simulink model "tp4_2"  (R2024b)
settings: Solver=FixedStepAuto  StartTime=0.0  StopTime=500  FixedStep=0.1  RelTol=1e-3
values from neighbouring files (symbols this model uses):
  F_in = 0.0035    [codigo_profe.m]    (also in directo.m; directo2.m; discretization.m; efecto_integral.m)
  F_out_sin_k = a*sqrt(2*g)    [tp4_inicio.m]
  h_list = [0.2, 0.4, 0.6, 0.8]    [tp4_inicio.m]
  k_list = [0.05, 0.15, 0.30, 0.50, 0.90]    [directo.m]    (also in directo2.m; discretization.m; efecto_integral.m; indirecto.m)
  r_0 = 0.05    [codigo_profe.m]    (also in directo.m; directo2.m; discretization.m; efecto_integral.m)
  theta = 60    [codigo_profe.m]    (also in directo.m; directo2.m; discretization.m; efecto_integral.m)
undefined symbols (not defined in the file or in its folder): A, B, C, D
libraries: ctrlSharedLib x1, simulink x1
settings Model: Creator=trulscarlson  LastModifiedBy=trulscarlson
settings DebuggingCC: UnconnectedInputMsg=warning  UnconnectedOutputMsg=warning  UnconnectedLineMsg=warning
settings ModelReferenceCC: EnableRefExpFcnMdlSchedulingChecks=on
settings RTWCC: GPUComputeCapability=3.5  DLArmComputeVersion=19.05

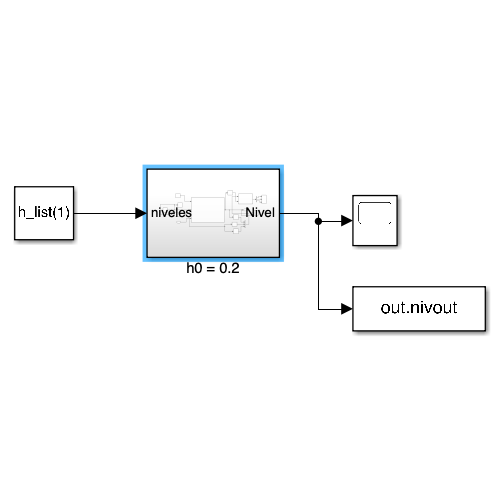
[thumbnail: Simulink's stored preview of the top-level diagram]
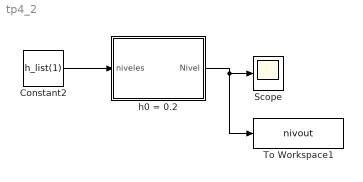
== system tp4_2 ==
  Constant2 : Constant  Value=h_list(1)
  Scope : Scope
  To Workspace1 : ToWorkspace  VariableName=nivout  SaveFormat=Timeseries  SampleTime=-1
  h0 = 0.2 : Subsystem
  wires:
  Constant2/1 -> h0 = 0.2/1(niveles)
  h0 = 0.2/1(Nivel) -> To Workspace1/1, Scope/1

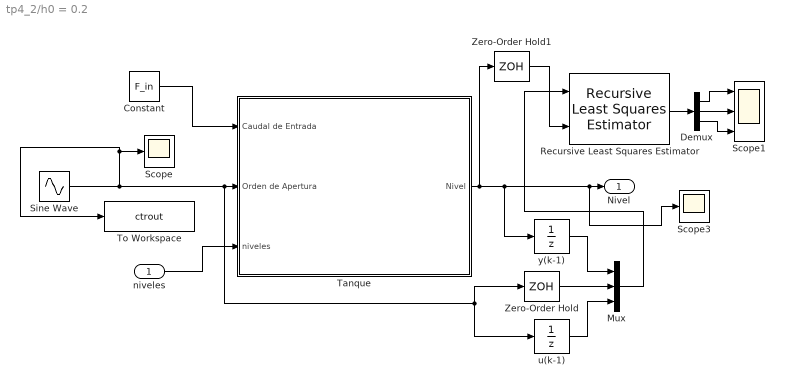
== system tp4_2/h0 = 0.2 ==
  niveles : Inport
  Constant : Constant  Value=F_in
  Demux : Demux  Outputs=3
  Mux : Mux  Inputs=3
  Recursive Least Squares Estimator : ctrlSharedLib/Recursive Least Squares Estimator  InitialEstimateSource=Internal  InitialParameterData=[0 0 0]  P0=1e5  InitialRegressors=0  InitialOutputs=0  History=Infinite  WindowLength=200  EstimationMethod=Forgetting Factor  AdaptationParameter=0.99  HasTimeVaryingAdaptationParameter=off  NormalizationBias=eps  OutputError=off  OutputP=off  AddEnablePort=off  InputProcessing=Sample-based  Ts=-1
      settings: LibrarySourceBlock=slident/Estimators/Recursive Least Squares Estimator
  Scope : Scope
  Scope1 : Scope  NumInputPorts=3
  Scope3 : Scope
  Sine Wave : Sin  Amplitude=0.2  Bias=k_list(1)  SampleTime=0
  Tanque : Subsystem
  To Workspace : ToWorkspace  VariableName=ctrout  SaveFormat=Timeseries  SampleTime=-1
  Zero-Order Hold : ZeroOrderHold  SampleTime=-1
  Zero-Order Hold1 : ZeroOrderHold  SampleTime=-1
  u(k-1) : UnitDelay  InitialCondition=k_list(1)  SampleTime=-1  HasFrameUpgradeWarning=on
  y(k-1) : UnitDelay  InitialCondition=h_list(1)  SampleTime=-1  HasFrameUpgradeWarning=on
  Nivel : Outport
  wires:
  niveles/1 -> Tanque/3(niveles)
  Constant/1 -> Tanque/1(Caudal de Entrada)
  Tanque/1(Nivel) -> Zero-Order Hold1/1, Scope3/1, Nivel/1, y(k-1)/1
  Sine Wave/1 -> Scope/1, To Workspace/1, u(k-1)/1, Zero-Order Hold/1, Tanque/2(Orden de Apertura)
  y(k-1)/1 -> Mux/1
  u(k-1)/1 -> Mux/3
  Mux/1 -> Recursive Least Squares Estimator/1
  Zero-Order Hold/1 -> Mux/2
  Zero-Order Hold1/1 -> Recursive Least Squares Estimator/2
  Recursive Least Squares Estimator/1 -> Demux/1
  Demux/1 -> Scope1/1
  Demux/2 -> Scope1/2
  Demux/3 -> Scope1/3

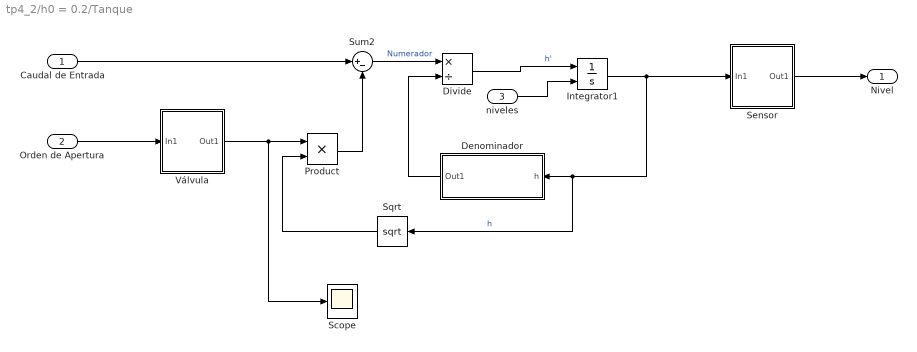
== system tp4_2/h0 = 0.2/Tanque ==
  Caudal de Entrada : Inport
  Orden de Apertura : Inport  Port=2
  niveles : Inport  Port=3
  Denominador : Subsystem
  Divide : Product  Inputs=*/
  Integrator1 : Integrator  InitialConditionSource=external  InitialCondition=h_list(5)
  Product : Product
  Scope : Scope
  Sensor : Subsystem
  Sqrt : Sqrt
  Sum2 : Sum  Inputs=|+-
  Válvula : Subsystem
  Nivel : Outport
  wires:
  Product/1 -> Sum2/2
  Divide/1 -> Integrator1/1  "h'"
  Denominador/1(Out1) -> Divide/2
  Integrator1/1 -> Sensor/1(In1), Sqrt/1, Denominador/1(h)  "h"
  Sum2/1 -> Divide/1  "Numerador"
  Sqrt/1 -> Product/2
  Caudal de Entrada/1 -> Sum2/1
  Orden de Apertura/1 -> Válvula/1(In1)
  Válvula/1(Out1) -> Product/1, Scope/1
  niveles/1 -> Integrator1/2
  Sensor/1(Out1) -> Nivel/1

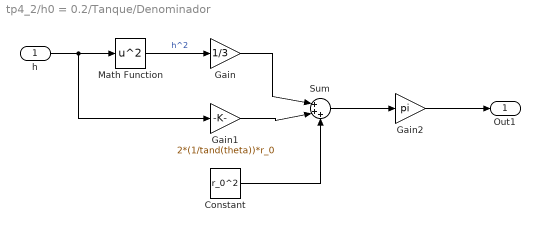
== system tp4_2/h0 = 0.2/Tanque/Denominador ==
  h : Inport
  Constant : Constant  Value=r_0^2
  Gain : Gain  Gain=1/3
  Gain1 : Gain  Gain=2*(1/tand(theta))*r_0
  Gain2 : Gain  Gain=pi
  Math Function : Math  Operator=square
  Sum : Sum  Inputs=|+++
  Out1 : Outport
  wires:
  h/1 -> Gain1/1, Math Function/1
  Math Function/1 -> Gain/1  "h^2"
  Gain/1 -> Sum/1
  Gain1/1 -> Sum/2
  Constant/1 -> Sum/3
  Sum/1 -> Gain2/1
  Gain2/1 -> Out1/1

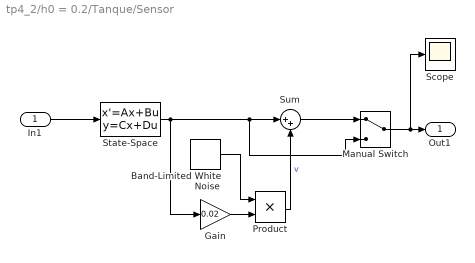
== system tp4_2/h0 = 0.2/Tanque/Sensor ==
  In1 : Inport
  Band-Limited White Noise : simulink/Sources/Band-Limited White Noise  Cov=[0.005]  Ts=0.1  seed=[23341]
  Gain : Gain  Gain=0.02
  Manual Switch : ManualSwitch
  Product : Product
  Scope : Scope
  State-Space : StateSpace  A=A  B=B  C=C  D=D  InitialCondition=h_list(1)*10
  Sum : Sum  Inputs=|++
  Out1 : Outport
  wires:
  In1/1 -> State-Space/1
  State-Space/1 -> Sum/1, Manual Switch/2, Gain/1
  Product/1 -> Sum/2  "v"
  Band-Limited White Noise/1 -> Product/1
  Gain/1 -> Product/2
  Sum/1 -> Manual Switch/1
  Manual Switch/1 -> Scope/1, Out1/1

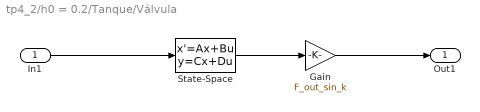
== system tp4_2/h0 = 0.2/Tanque/Válvula ==
  In1 : Inport
  Gain : Gain  Gain=F_out_sin_k
  State-Space : StateSpace  A=A  B=B  C=C  D=D  InitialCondition=k_list(1)*10
  Out1 : Outport
  wires:
  State-Space/1 -> Gain/1
  Gain/1 -> Out1/1
  In1/1 -> State-Space/1
